simulink model "c6416dsksurveil_hsrtdx"  (Simulink 6.0)
settings: Solver=FixedStepDiscrete  SolverMode=SingleTasking  StartTime=0.0  StopTime=inf  RelTol=1e-3
libraries: rtdxBlocks x5, c6416dsklib x2, dspsigops x2, dspmtrx3 x2, c6000tgtpreflib x1, simulink x1
CloseFcn:
  | clear vR3 vG3 vB3
settings Model: Creator=don  LastModifiedBy=thartley  ProdHWDeviceType=TI C6000
settings DataIOCC: LimitDataPoints=off  SaveOutput=off  SaveTime=off  SignalLoggingName=sigsOut
settings OptimizationCC: InlineInvariantSignals=off  EnforceIntegerDowncast=off
settings DebuggingCC: CheckExecutionContextPreStartOutputMsg=on  CheckExecutionContextRuntimeOutputMsg=on  SolverPrmCheckMsg=none
settings HardwareCC: ProdBitPerLong=40  ProdEndianess=LittleEndian  ProdHWDeviceType=TI C6000  TargetHWDeviceType=32-bit Generic
settings ModelReferenceCC: UpdateModelReferenceTargets=IfOutOfDate
settings RTWCC: SystemTargetFile=ti_c6000.tlc  TemplateMakefile=ti_c6000.tmf  ProcessScript=ti_c6000_make_rtw_hook
settings STFCustomTargetCC: TargetFcnLib=ansi_tfl_tmw.mat  MatFileLogging=on  LifeSpan=inf  SystemTargetFile=ti_c6000.tlc  ActivateCallback=c6000_callback('ActivateCallback',hSrc,hDlg);
settings GRTTargetCC: ModelReferenceCompliant=off  LifeSpan=inf
settings CustomProperty: DataType=RTWOptions_EnumType_S__A_matlab_toolbox_rtw_targets_tic6000_tic6000_ti_c6000_BoardType  Value=C6416DSK
settings EnumStrPairs: String=C6416DSK
settings SFSimCC: SFSimApplyToAllLibs=on  SFSimBuildMode=Incremental

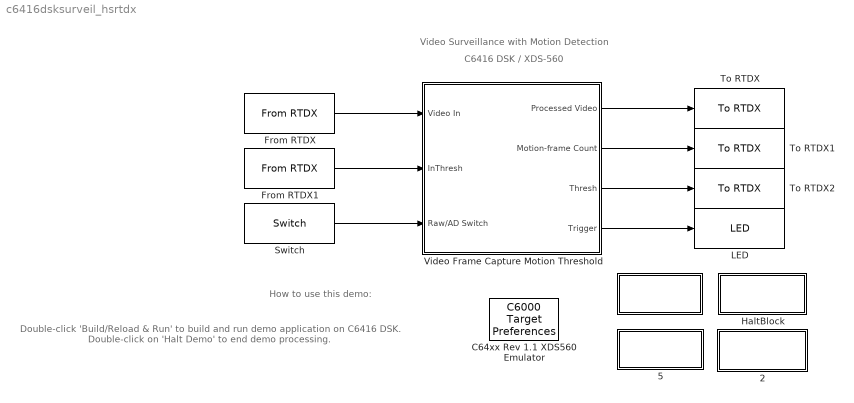
== system c6416dsksurveil_hsrtdx ==
  note: Video Surveillance with Motion Detection
  note: C6416 DSK / XDS-560
  note: Double-click 'Build/Reload & Run' to build and run
      | demo application on C6416 DSK.  Double-click
      | on 'Halt Demo' to end demo processing.
  note: How to use this demo:
  " " : Subsystem
      settings: OpenFcn=surveil_script('run')
      mask Type: Run demo
      mask Display: disp(sprintf('Build / Reload\n& Run'))
  " 2" : Subsystem
      settings: OpenFcn=edit surveil_script
      mask Type: Run demo
      mask Description: Double-clicking this button will display the demo script which generates code, builds, loads, executes application on the DSP, and arbitrates RTDX transfers.
      mask Display: disp(sprintf('View Demo \nScript'))
  " 5" : Subsystem
      settings: OpenFcn=web(fullfile(matlabroot,'toolbox','rtw','targets','tic6000','tic6000demos','html','VideoSurveillance_doc.html'))
      mask Type: Run demo
      mask Description: Double-clicking this button will display the demo script which generates code, builds, loads, executes application on the DSP, and arbitrates RTDX transfers.
      mask Display: disp('Info')
  C64xx Rev 1.1 XDS560 Emulator : c6000tgtpreflib/C6000 Target Preferences
  From RTDX : rtdxBlocks/From RTDX  channelNameStr=videoFrames  isBlocking=off  icMaskVar=0  Ts=1/15  dims=[120 160]  isFrame=off  dType=uint8  isChannelEnabled=on  isHighSpeedRTDXUsed=on
  From RTDX1 : rtdxBlocks/From RTDX  channelNameStr=motionThreshold  isBlocking=off  icMaskVar=1.5e5  Ts=1/15  dims=[1 1]  isFrame=off  dType=int32  isChannelEnabled=on  isHighSpeedRTDXUsed=on
  HaltBlock : Subsystem  Description=Terminates RTDX processing as necessary, and resets DSP.  AncestorBlock=c6711dsklib/Reset
      settings: OpenFcn=surveil_script('halt')
      mask Display: disp('Halt Demo');
  LED : c6416dsklib/LED
  Switch : c6416dsklib/Switch  sw0=off  sw1=off  sw2=off  sw3=off  dType=Boolean  Ts=1/15
  To RTDX : rtdxBlocks/To RTDX  channelNameStr=motionFrames  isChannelEnabled=on
  To RTDX1 : rtdxBlocks/To RTDX  channelNameStr=eventCnt  isChannelEnabled=on
  To RTDX2 : rtdxBlocks/To RTDX  channelNameStr=motionEst  isChannelEnabled=on
  Video Frame Capture Motion Threshold : Subsystem  TreatAsAtomicUnit=on
  wires:
  Video Frame Capture Motion Threshold/1(Processed Video) -> To RTDX/1
  Video Frame Capture Motion Threshold/2(Motion-frame Count) -> To RTDX1/1
  From RTDX/1 -> Video Frame Capture Motion Threshold/1(Video In)
  Video Frame Capture Motion Threshold/4(Trigger) -> LED/1
  Video Frame Capture Motion Threshold/3(Thresh) -> To RTDX2/1
  Switch/1 -> Video Frame Capture Motion Threshold/3(Raw/AD Switch)
  From RTDX1/1 -> Video Frame Capture Motion Threshold/2(InThresh)

== system c6416dsksurveil_hsrtdx/  ==

== system c6416dsksurveil_hsrtdx/ 2 ==

== system c6416dsksurveil_hsrtdx/ 5 ==

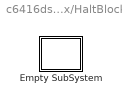
== system c6416dsksurveil_hsrtdx/HaltBlock ==
  Empty SubSystem : Subsystem

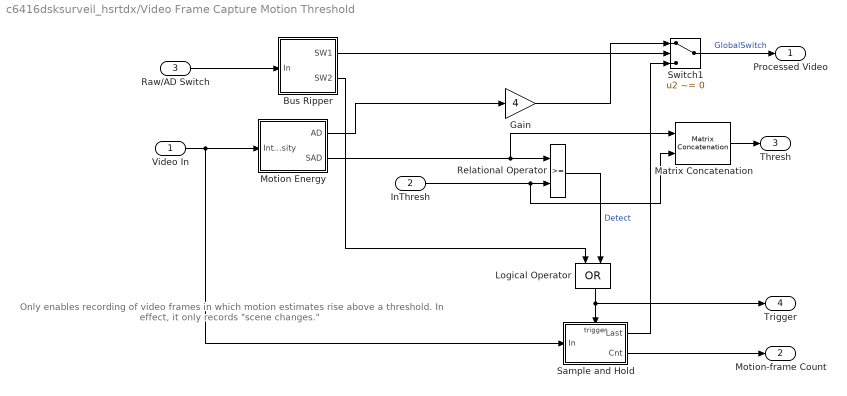
== system c6416dsksurveil_hsrtdx/Video Frame Capture Motion Threshold ==
  note: Only enables recording of video frames in
      | which motion estimates rise above a threshold.
      | In effect, it only records "scene changes."
  Video In : Inport
  InThresh : Inport  Port=2
  Raw/AD Switch : Inport  Port=3
  Bus Ripper : Subsystem
  Gain : Gain  Gain=4  ParameterDataType=uint(8)  OutDataTypeMode=Specify via dialog  OutDataType=uint(8)  SaturateOnIntegerOverflow=on
  Logical Operator : Logic  Orientation=down  Operator=OR  AllPortsSameDT=off
  Matrix Concatenation : simulink/Math Operations/Matrix Concatenation  numInports=2  catMethod=Vertical
  Motion Energy : Subsystem
  Relational Operator : RelationalOperator  LogicOutDataTypeMode=Boolean  InputSameDT=on
  Sample and Hold : Subsystem  AncestorBlock=dspsigops/Sample and Hold  TreatAsAtomicUnit=on  mask(Sample and Hold){trig=Either edge, initCond=0}
      mask prompts: trig "Trigger type:"; initCond "Initial condition:"
      mask help: Sample and hold input signal.
      mask init:
      | switch trig
      | case 1, s='rising';
      | case 2, s='falling';
      | case 3, s='either';
      | end
      | set_param([gcb '/Trigger'],'triggertype',s);
      mask Help: web(dspbhelp);
      mask StyleString: popup(Rising edge|Falling edge|Either edge),edit
      mask Display: disp('S/H')
  Switch1 : Switch  Criteria=u2 ~= 0  ZeroCross=off
  Processed Video : Outport
  Motion-frame Count : Outport  Port=2
  Thresh : Outport  Port=3
  Trigger : Outport  Port=4
  wires:
  Matrix Concatenation/1 -> Thresh/1
  Video In/1 -> Sample and Hold/1(In), Motion Energy/1(Intensity)
  Bus Ripper/1(SW1) -> Switch1/2
  Motion Energy/2(SAD) -> Matrix Concatenation/1, Relational Operator/1
  Motion Energy/1(AD) -> Gain/1
  Gain/1 -> Switch1/1
  Sample and Hold/1(Last) -> Switch1/3
  InThresh/1 -> Matrix Concatenation/2, Relational Operator/2
  Switch1/1 -> Processed Video/1  "GlobalSwitch"
  Sample and Hold/2(" Cnt") -> Motion-frame Count/1
  Bus Ripper/2(SW2) -> Logical Operator/1
  Relational Operator/1 -> Logical Operator/2  "Detect"
  Logical Operator/1 -> Sample and Hold/Trigger, Trigger/1
  Raw/AD Switch/1 -> Bus Ripper/1(In)

== system c6416dsksurveil_hsrtdx/HaltBlock/Empty SubSystem ==

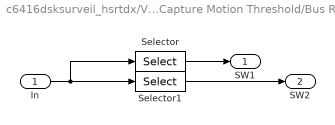
== system c6416dsksurveil_hsrtdx/Video Frame Capture Motion Threshold/Bus Ripper ==
  In : Inport
  Selector : Selector  InputPortWidth=4
  Selector1 : Selector  Elements=2  InputPortWidth=4
  SW1 : Outport
  SW2 : Outport  Port=2
  wires:
  In/1 -> Selector/1, Selector1/1
  Selector/1 -> SW1/1
  Selector1/1 -> SW2/1

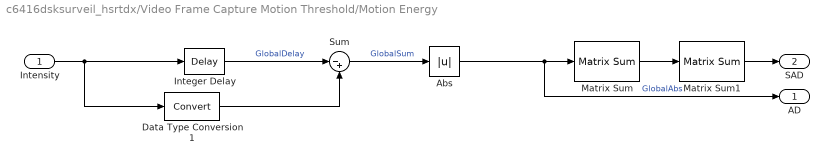
== system c6416dsksurveil_hsrtdx/Video Frame Capture Motion Threshold/Motion Energy ==
  Intensity : Inport
  Abs : Abs  SaturateOnIntegerOverflow=on
  Data Type Conversion1 : DataTypeConversion  OutDataTypeMode=int16  RndMeth=Zero
  Integer Delay : dspsigops/Delay  delay=1  ic=0  reset_popup=None
  Matrix Sum : dspmtrx3/Matrix Sum  Dim=Columns  outputMode=User-defined  outputWordLength=32  outputFracLength=0  roundingMode=Floor  overflowMode=off
      settings: additionalParams=on
  Matrix Sum1 : dspmtrx3/Matrix Sum  Dim=Rows  roundingMode=Floor  overflowMode=off
  Sum : Sum  Inputs=|-+
  AD : Outport
  SAD : Outport  Port=2
  wires:
  Intensity/1 -> Integer Delay/1, Data Type Conversion1/1
  Sum/1 -> Abs/1  "GlobalSum"
  Integer Delay/1 -> Sum/1  "GlobalDelay"
  Abs/1 -> AD/1, Matrix Sum/1  "GlobalAbs"
  Matrix Sum1/1 -> SAD/1
  Data Type Conversion1/1 -> Sum/2
  Matrix Sum/1 -> Matrix Sum1/1

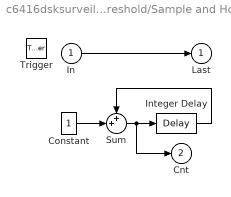
== system c6416dsksurveil_hsrtdx/Video Frame Capture Motion Threshold/Sample and Hold ==
  In : Inport
  Trigger : TriggerPort  TriggerType=either  StatesWhenEnabling=reset  ZeroCross=off
  Constant : Constant  OutDataTypeMode=int32
  Integer Delay : dspsigops/Delay  delay=1  ic=0  reset_popup=None
  Sum : Sum  Inputs=++|
  Last : Outport  InitialOutput=initCond
  " Cnt" : Outport  Port=2
  wires:
  In/1 -> Last/1
  Constant/1 -> Sum/2
  Sum/1 -> Integer Delay/1, " Cnt"/1
  Integer Delay/1 -> Sum/1
